simulink model "onduleur"  (R2013a)
settings: Solver=ode45  StartTime=0.0  StopTime=0.06  RelTol=1e-3
libraries: powerlib x10, dspstat3 x1
settings Model: Creator=DELL  LastModifiedBy=DELL

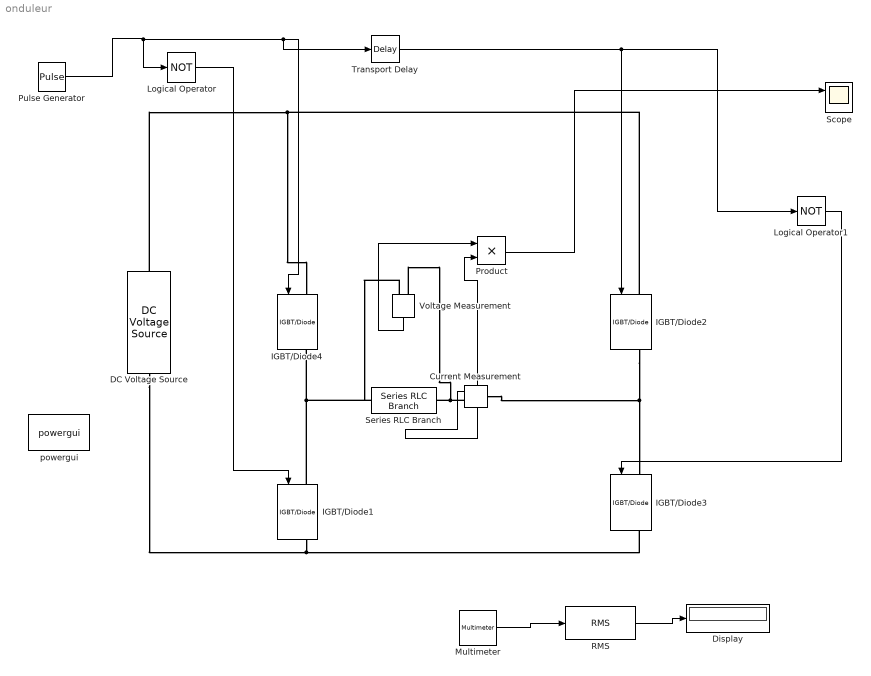
== system onduleur ==
  Current Measurement : powerlib/Measurements/Current Measurement  PhasorSimulation=off  OutputType=Complex  PSBequivalent=0
  DC Voltage Source : powerlib/Electrical Sources/DC Voltage Source  Amplitude=100  Measurements=None
  Display : Display
  IGBT/Diode{1..4} (4 alike) : powerlib/Power Electronics/IGBT//Diode  Ron=1e-3  Rs=1e5  Cs=inf  Measurements=on
  Logical Operator : Logic  Operator=NOT  AllPortsSameDT=off  OutDataTypeStr=boolean
  Logical Operator1 : Logic  Operator=NOT  AllPortsSameDT=off  OutDataTypeStr=boolean
  Multimeter : powerlib/Measurements/Multimeter  PhasorSimulation=off  OutputType=Complex  sel=[1 2]  L=2  Gain=[1 1]  yselected={'Ub: Series RLC Branch','Ib: Series RLC Branch'};  PSBOutputType=1  PSBequivalent=0  AxesSetting=[0,0.1,-100,100]  Display=1  SavedBlockNames=-11
  Product : Product
  Pulse Generator : DiscretePulseGenerator  PulseType=Time based  Amplitude=5  Period=0.02  PulseWidth=50
  RMS : dspstat3/RMS  run=off  reset_popup=None  InputProcessing=Columns as channels (frame based)  directionMode=Each column  dimension=1  treatSBRowAsCol=on
  Scope : Scope  NumInputPorts=2
      settings: YMin=-5~-5  YMax=5~5
  Series RLC Branch : powerlib/Elements/Series RLC Branch  LConnTagsString=__new0  RConnTagsString=__new0  BranchType=R  Resistance=10  Inductance=0.02  SetiL0=off  InitialCurrent=0  Capacitance=1e-6  Setx0=off  InitialVoltage=0  Measurements=Branch voltage and current
  Transport Delay : TransportDelay  DelayTime=0.005
  Voltage Measurement : powerlib/Measurements/Voltage Measurement  PhasorSimulation=off  OutputType=Complex  PSBequivalent=0
  powergui : powerlib/powergui  Priority=1  SimulationMode=Continuous  SolverType=Tustin  SampleTime=50e-6  frequency=60  SPID=off  DisableSnubberDevices=off  DisableRonSwitches=off  DisableVfSwitches=off  SwTol=0  Interpol=off  DisplayEquations=off  frequencyindice=0  Pbase=100e6  ErrMax=1e-4  Iterations=50  UnitsV=kV  UnitsW=MW  FunctionMessages=off  echomessages=off  HookPort=off  EnableUseOfTLC=off  x0status=blocks  RestoreLinks=warning  ResistiveCurrentMeasurement=off  Frange=[0:2:500]  Ylog=off  Xlog=on  ShowGrid=off  save=off  variable=ZData  ZoomFFT=off  StartTime=0.0  cycles=1  DisplayStyle=1  fundamental=60  FreqAxis=off  MaxFrequency=1000  frequencyindicesteady=1  RmsSteady=1  display=off  Ts=0  methode=off
  wires:
  RMS/1 -> Display/1
  Multimeter/1 -> RMS/1
  Logical Operator/1 -> IGBT/Diode1/1
  Current Measurement/1 -> Product/2
  Voltage Measurement/1 -> Product/1
  Product/1 -> Scope/1
  Transport Delay/1 -> IGBT/Diode2/1, Logical Operator1/1
  Logical Operator1/1 -> IGBT/Diode3/1
  Pulse Generator/1 -> IGBT/Diode4/1, Transport Delay/1, Logical Operator/1
  connections:
  IGBT/Diode2/LConn1 -- DC Voltage Source/RConn1 -- IGBT/Diode4/LConn1
  IGBT/Diode1/LConn1 -- Voltage Measurement/LConn1 -- Series RLC Branch/LConn1 -- IGBT/Diode4/RConn1
  IGBT/Diode2/RConn1 -- Current Measurement/LConn1 -- IGBT/Diode3/LConn1
  DC Voltage Source/LConn1 -- IGBT/Diode1/RConn1 -- IGBT/Diode3/RConn1
  Current Measurement/RConn1 -- Voltage Measurement/LConn2 -- Series RLC Branch/RConn1
